simulink model "Los_path_old"  (R2023b)
settings: Solver=VariableStepAuto  StartTime=0.0  StopTime=200  RelTol=1e-3
values from neighbouring files (symbols this model uses):
  current = [0, 0, 0, 0]'    [Los_path_mat.m]
  deltah = 4    [Los_path_mat.m]
  depth_des = 0.5    [Los_path_mat.m]
  des_vel = [0.1, 0, 0, 0]'    [Kal_6Dpitch_mat.m]    (also in Los_path_mat.m)
  eta_init = [0.1, 0, 0, 0.7]'    [Los_path_mat.m]
  Kd_dep = (p + 2*damp*wn)*mv(3) + dv(3)    [Control_gains_mat.m]    (also in Los_path_mat.m = (p + 2*damp*wn)*mv(4) + dv(4))
  Kd_yaw = (p + 2*damp*wn)*mv(3) - dv(3)    [Los_path_mat.m]
  Ki_dep = p*(wn^2)*mv(3)    [Control_gains_mat.m]    (also in Los_path_mat.m = p*(wn^2)*mv(4))
  Ki_surge = wn^2 * mv(1)    [Control_gains_mat.m]    (also in Los_path_mat.m)
  Ki_yaw = p*(wn^2)*mv(3)    [Los_path_mat.m]
  Kp_dep = mv(3)*((wn^2) + 2*damp*p*wn)    [Control_gains_mat.m]    (also in Los_path_mat.m = mv(4)*((wn^2) + 2*damp*p*wn))
  Kp_surge = 2*damp*wn*mv(1) - dv(1)    [Control_gains_mat.m]    (also in Los_path_mat.m)
  Kp_yaw = mv(3)*((wn^2) + 2*damp*p*wn)    [Los_path_mat.m]
  speed0 = [0.1, 0, 0, 0]'    [Los_path_mat.m]    (also in Model_6Deq_mat.m = [0.1, 0, 0, 0, 0, 0]')
libraries: simulink x2
settings Model: Creator=fabio  LastModifiedBy=fabio

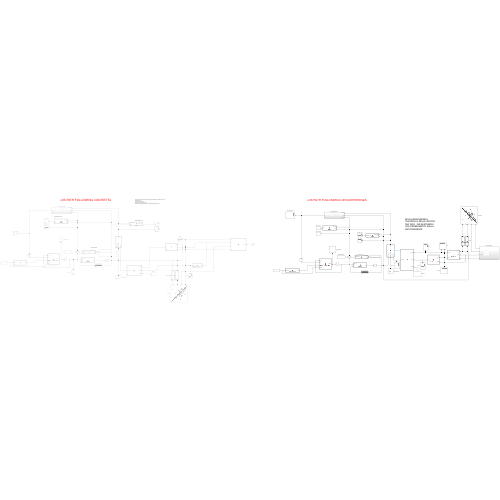
[thumbnail: Simulink's stored preview of the top-level diagram]
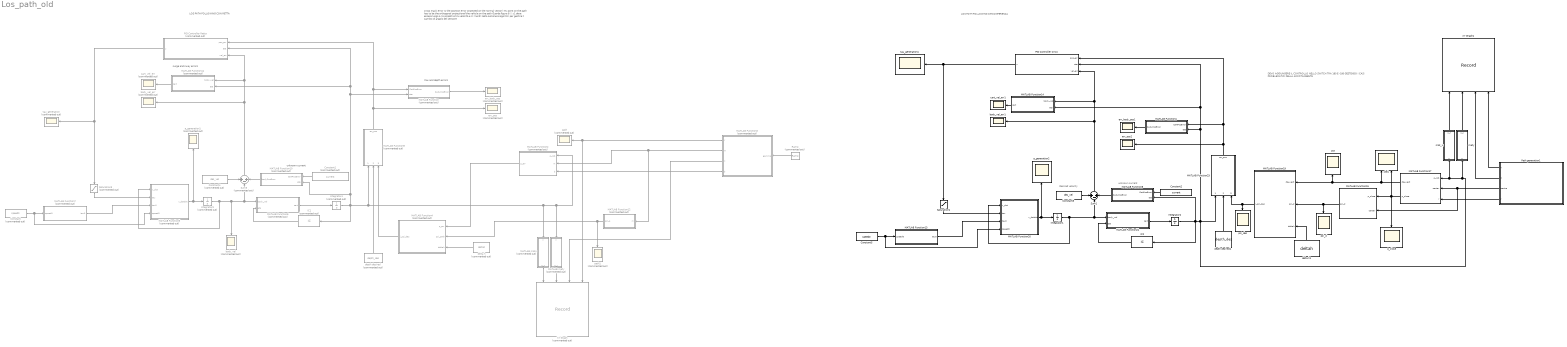
== system Los_path_old ==
  note: cross track error is the position error projected on the normal vector)
      | My point on the path has to be the orthogonal projectionof the vehicle on the path
      | Guarda figura 8 !!
      | y1 deve essere lungo a n1
      | psipath è tra velocità e Xi (nord)
      | Nella sezione 6 algoritm per gestire il cambio di angolo del sensore
  note: surge and sway errors
  note: Yaw and depth errors
  note: DEVO AGGIUNGERE IL CONTROLLO NELLO SWITCH TRA 180 E -180 GESTENDO I CASI PROBLEMATICI DELLA ARCOTANGENTE
  note: Desired velocity
  note: unknown current
  note: LOS PATH FOLLOWING CON RETTA
  note: unknown current
  note: LOS PATH FOLLOWING CIRCONFERENZA
  Constant : Constant  Commented=on  Value=speed0
  Constant1 : Constant  Commented=on  Value=current
  Constant2 : Constant  Value=current
  Constant3 : Constant  Value=des_vel
  Constant4 : Constant  Commented=on  Value=des_vel
  Constant5 : Constant  Value=speed0
  IC1 : InitialCondition  Commented=on  Value=eta_init
  IC2 : InitialCondition  Value=eta_init
  Integrator1 : Integrator
  Integrator2 : Integrator
  Integrator3 : Integrator  Commented=on
  Integrator4 : Integrator  Commented=on
  MATLAB Function : MATLAB Function  Commented=on  TreatAsAtomicUnit=on
  MATLAB Function1 : MATLAB Function  TreatAsAtomicUnit=on
  MATLAB Function10 : MATLAB Function  Commented=on  TreatAsAtomicUnit=on
  MATLAB Function11 : MATLAB Function  Commented=on  TreatAsAtomicUnit=on
  MATLAB Function12 : MATLAB Function  Commented=on  TreatAsAtomicUnit=on
  MATLAB Function13 : MATLAB Function  TreatAsAtomicUnit=on
  MATLAB Function14 : MATLAB Function  TreatAsAtomicUnit=on
  MATLAB Function15 : MATLAB Function  TreatAsAtomicUnit=on
  MATLAB Function17 : MATLAB Function  TreatAsAtomicUnit=on
  MATLAB Function19 : MATLAB Function  TreatAsAtomicUnit=on
  MATLAB Function2 : MATLAB Function  Commented=on  TreatAsAtomicUnit=on
  MATLAB Function20 : MATLAB Function  TreatAsAtomicUnit=on
  MATLAB Function21 : MATLAB Function  TreatAsAtomicUnit=on
  MATLAB Function23 : MATLAB Function  TreatAsAtomicUnit=on
  MATLAB Function3 : MATLAB Function  Commented=on  TreatAsAtomicUnit=on
  MATLAB Function4 : MATLAB Function  Commented=on  TreatAsAtomicUnit=on
  MATLAB Function5 : MATLAB Function  Commented=on  TreatAsAtomicUnit=on
  MATLAB Function6 : MATLAB Function  Commented=on  TreatAsAtomicUnit=on
  MATLAB Function7 : MATLAB Function  Commented=on  TreatAsAtomicUnit=on
  MATLAB Function8 : MATLAB Function  TreatAsAtomicUnit=on
  MATLAB Function9 : MATLAB Function  Commented=on  TreatAsAtomicUnit=on
  MATLAB matx : MATLAB Function  Commented=on  TreatAsAtomicUnit=on
  MATLAB maty : MATLAB Function  Commented=on  TreatAsAtomicUnit=on
  PID Controller Circo : Subsystem
  PID Controller Retta : Subsystem  Commented=on
  Path generation1 : Subsystem
  Ramp : simulink/Sources/Ramp  Commented=on  slope=1  start=0  InitialOutput=0
  Saturation1 : Saturate  UpperLimit=20000  LowerLimit=-20000
  Saturation3 : Saturate  Commented=on  UpperLimit=20000  LowerLimit=-20000
  Sum1 : Sum  Inputs=+-+
  Sum5 : Sum  Commented=on  Inputs=+-+
  XY Graph : Record  Commented=on  FileSettingsInternal="{\"entries\":[{\"content\":{\"excelSettings\":{\"content\":{},\"type\":\"Streamout.ExcelSettings\"}},\"type\":\"Streamout.FileSettingStorage\",\"uuid\":\"\"}],\"packageUris\":[\"http:\\/\\/schema.mathworks.com\\/mf0\\/streamout_blocks\\/R2020a\"],\"version\":\"1.0\"}"  Layout=[1 1]  SignalsInternal="{\"entries\":[{\"content\":{},\"type\":\"RecordBlkView.InputSignals\",\"uuid\":\"\"}],\"packageUris\":[\"http:\\/\\/schema.mathworks.com\\/mf0\\/streamout_blocks\\/R2020a\"],\"version\":\"1.0\"}"  VisualizationBindings="{\"xyplotplugin\":{\"info\":[{\"series\":[],\"subplotID\":1}]}}"  CompatibilityTag=XY
  XY Graph1 : Record  FileSettingsInternal="{\"entries\":[{\"content\":{\"excelSettings\":{\"content\":{},\"type\":\"Streamout.ExcelSettings\"}},\"type\":\"Streamout.FileSettingStorage\",\"uuid\":\"\"}],\"packageUris\":[\"http:\\/\\/schema.mathworks.com\\/mf0\\/streamout_blocks\\/R2020a\"],\"version\":\"1.0\"}"  Layout=[1 1]  SignalsInternal="{\"entries\":[{\"content\":{},\"type\":\"RecordBlkView.InputSignals\",\"uuid\":\"\"}],\"packageUris\":[\"http:\\/\\/schema.mathworks.com\\/mf0\\/streamout_blocks\\/R2020a\"],\"version\":\"1.0\"}"  VisualizationBindings="{\"xyplotplugin\":{\"info\":[{\"series\":[],\"subplotID\":1}]}}"  CompatibilityTag=XY
  a_generation1 : Scope  Commented=on
  a_generation2 : Scope
  body_vel : Scope  Commented=on
  body_vel_err : Scope  Commented=on
  body_vel_err1 : Scope
  cart_vel_err : Scope  Commented=on
  cart_vel_err1 : Scope
  cte : Scope
  cte1 : Scope  NumInputPorts=2
  delta h : Constant  Commented=on  Value=deltah
  delta h1 : Constant  Value=deltah
  depth desired : Constant  Commented=on  Value=depth_des
  depth desired1 : Constant  Value=depth_des
  err_body_pos : Scope  Commented=on
  err_body_pos1 : Scope
  err_pos : Scope  Commented=on
  err_pos2 : Scope
  mat_x : MATLAB Function  TreatAsAtomicUnit=on
  maty : MATLAB Function  TreatAsAtomicUnit=on
  p_close : Scope
  path : Scope  Commented=on
  path1 : Scope  Commented=on
  psi_d : Scope
  psi_des : Scope
  tau_generation : Scope  Commented=on
  tau_generation1 : Scope
  wires:
  PID Controller Retta/1(u) -> Saturation3/1, tau_generation/1
  Integrator3/1 -> body_vel/1, MATLAB Function6/1(body_vel), Sum5/2, MATLAB Function5/1(x_dot)
  Saturation3/1 -> MATLAB Function5/2(tau)
  MATLAB Function7/1(tau0) -> MATLAB Function5/3(tau0)
  MATLAB Function5/1(x_dotdot) -> Integrator3/1, a_generation1/1
  MATLAB Function6/1(cart) -> Integrator4/1
  IC1/1 -> MATLAB Function6/2(eta)
  MATLAB Function/1(bodyPosError) -> err_body_pos/1
  Sum5/1 -> PID Controller Retta/3(vel_err), MATLAB Function11/1(body_vel), body_vel_err/1
  Ramp/1 -> MATLAB Function3/1(gamma)
  MATLAB Function3/1(Y) -> path/1, XY Graph/4
  MATLAB Function3/2(m) -> MATLAB Function12/1(m), MATLAB Function2/2(m)
  MATLAB Function3/4(b) -> MATLAB Function2/3(b)
  Constant4/1 -> Sum5/1
  Integrator4/1 -> MATLAB Function9/1(p_pose_err), MATLAB Function2/1(p_rob), MATLAB maty/1(u), MATLAB matx/1(u), MATLAB Function/2(eta), PID Controller Retta/2(eta), MATLAB Function11/2(eta), MATLAB Function10/2(eta), IC1/1
  MATLAB Function4/1(i_psi_des) -> MATLAB Function9/3(psi_path)
  MATLAB Function9/1(err_pos) -> PID Controller Retta/1(pos_err), MATLAB Function/1(CartPosError), err_pos/1
  depth desired/1 -> MATLAB Function9/2(depth_des)
  MATLAB Function11/1(cart) -> cart_vel_err/1
  MATLAB matx/1(u_x) -> XY Graph/1
  MATLAB maty/1(u_y) -> XY Graph/2
  MATLAB Function3/3(X) -> XY Graph/3
  MATLAB Function12/1(psi_p) -> path1/1, MATLAB Function4/2(psi_path)
  MATLAB Function2/1(p_err) -> MATLAB Function4/1(p_err)
  delta h/1 -> MATLAB Function4/3(deltah)
  MATLAB Function21/1(cart) -> Integrator2/1
  Sum1/1 -> PID Controller Circo/3(vel_err), MATLAB Function14/1(body_vel), body_vel_err1/1
  depth desired1/1 -> MATLAB Function23/2(depth_des)
  MATLAB Function14/1(cart) -> cart_vel_err1/1
  MATLAB Function23/1(err_pos) -> err_pos2/1, PID Controller Circo/1(pos_err), MATLAB Function1/1(CartPosError)
  Integrator1/1 -> MATLAB Function21/1(body_vel), Sum1/2, MATLAB Function20/1(x_dot)
  Constant3/1 -> Sum1/1
  MATLAB Function20/1(x_dotdot) -> Integrator1/1, a_generation2/1
  Integrator2/1 -> MATLAB Function8/2(eta), maty/1(u), mat_x/1(u), MATLAB Function17/1(p_rob), MATLAB Function14/2(eta), PID Controller Circo/2(eta), MATLAB Function1/2(eta), MATLAB Function23/1(p_pose_err), IC2/1
  MATLAB Function19/1(i_psi_des) -> MATLAB Function23/3(psi_path), psi_des/1
  MATLAB Function1/1(bodyPosError) -> err_body_pos1/1
  Saturation1/1 -> MATLAB Function20/2(tau)
  PID Controller Circo/1(u) -> Saturation1/1, tau_generation1/1
  IC2/1 -> MATLAB Function21/2(eta)
  Path generation1/3(centre) -> MATLAB Function15/2(center), MATLAB Function17/2(center)
  Path generation1/4(r) -> MATLAB Function17/3(r)
  MATLAB Function17/2(p_close) -> p_close/1, MATLAB Function15/1(p_close), cte1/2
  MATLAB Function15/1(psi_d) -> psi_d/1, MATLAB Function19/2(psi_d)
  MATLAB Function17/1(cte_vect) -> MATLAB Function19/1(cte_vect), cte/1, cte1/1
  delta h1/1 -> MATLAB Function19/3(deltah)
  Path generation1/2(X) -> XY Graph1/3
  Path generation1/1(Y) -> XY Graph1/4
  mat_x/1(u_x) -> XY Graph1/1
  maty/1(u_y) -> XY Graph1/2
  Constant2/1 -> MATLAB Function8/1(CartPosError)
  MATLAB Function8/1(bodyPosError) -> Sum1/3
  MATLAB Function10/1(bodyPosError) -> Sum5/3
  Constant1/1 -> MATLAB Function10/1(CartPosError)
  Constant/1 -> MATLAB Function5/4(speed0), MATLAB Function7/1(speed0)
  MATLAB Function13/1(tau0) -> MATLAB Function20/3(tau0)
  Constant5/1 -> MATLAB Function20/4(speed0), MATLAB Function13/1(speed0)

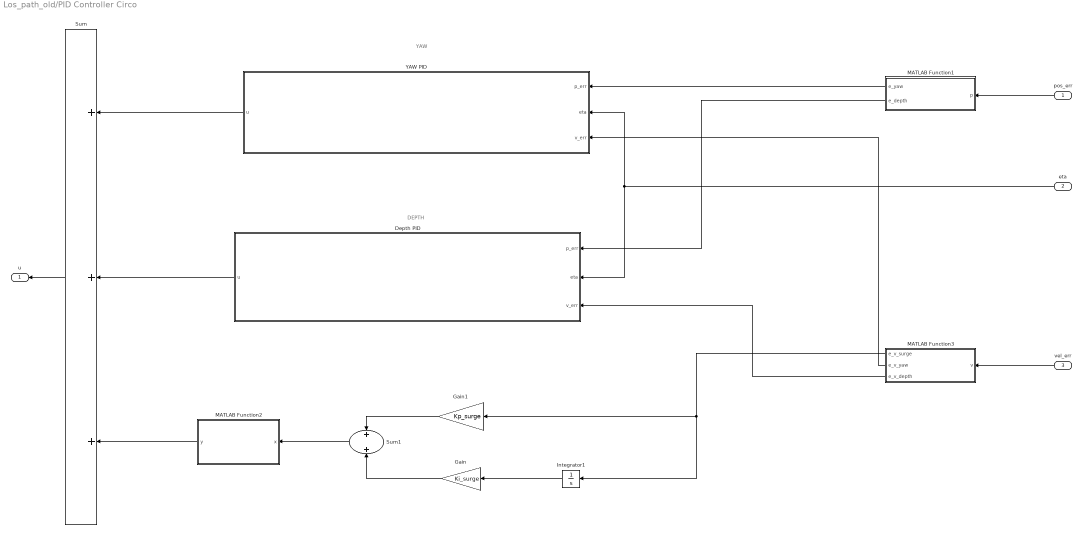
== system Los_path_old/PID Controller Circo ==
  note: YAW
  note: DEPTH
  pos_err : Inport
  eta : Inport  Port=2
  vel_err : Inport  Port=3
  Depth PID : Subsystem
  Gain : Gain  Gain=Ki_surge
  Gain1 : Gain  Gain=Kp_surge
  Integrator1 : Integrator
  MATLAB Function1 : MATLAB Function  TreatAsAtomicUnit=on
  MATLAB Function2 : MATLAB Function  TreatAsAtomicUnit=on
  MATLAB Function3 : MATLAB Function  TreatAsAtomicUnit=on
  Sum : Sum  Inputs=+++
  Sum1 : Sum
  YAW PID : Subsystem
  u : Outport
  wires:
  vel_err/1 -> MATLAB Function3/1(v)
  pos_err/1 -> MATLAB Function1/1(p)
  MATLAB Function1/2(e_depth) -> Depth PID/1(p_err)
  Integrator1/1 -> Gain/1
  Gain1/1 -> Sum1/1
  Sum/1 -> u/1
  YAW PID/1(u) -> Sum/1
  MATLAB Function1/1(e_yaw) -> YAW PID/1(p_err)
  Depth PID/1(u) -> Sum/2
  Gain/1 -> Sum1/2
  MATLAB Function3/1(e_v_surge) -> Gain1/1, Integrator1/1
  MATLAB Function3/2(e_v_yaw) -> YAW PID/3(v_err)
  MATLAB Function3/3(e_v_depth) -> Depth PID/3(v_err)
  Sum1/1 -> MATLAB Function2/1(x)
  eta/1 -> YAW PID/2(eta), Depth PID/2(eta)
  MATLAB Function2/1(y) -> Sum/3

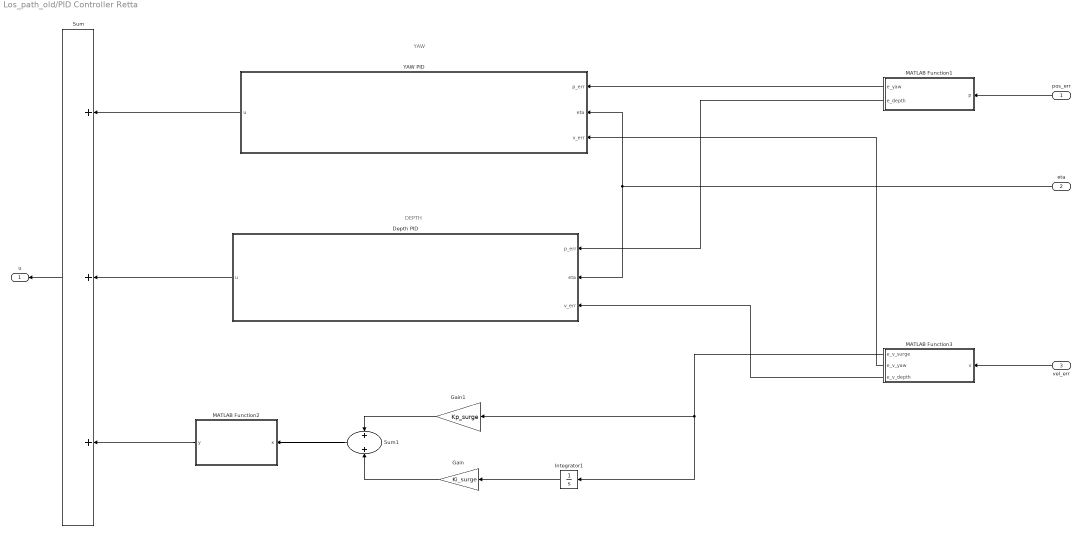
== system Los_path_old/PID Controller Retta ==
  note: DEPTH
  note: YAW
  pos_err : Inport
  eta : Inport  Port=2
  vel_err : Inport  Port=3
  Depth PID : Subsystem
  Gain : Gain  Gain=Ki_surge
  Gain1 : Gain  Gain=Kp_surge
  Integrator1 : Integrator
  MATLAB Function1 : MATLAB Function  TreatAsAtomicUnit=on
  MATLAB Function2 : MATLAB Function  TreatAsAtomicUnit=on
  MATLAB Function3 : MATLAB Function  TreatAsAtomicUnit=on
  Sum : Sum  Inputs=+++
  Sum1 : Sum
  YAW PID : Subsystem
  u : Outport
  wires:
  eta/1 -> YAW PID/2(eta), Depth PID/2(eta)
  Integrator1/1 -> Gain/1
  Sum1/1 -> MATLAB Function2/1(x)
  Sum/1 -> u/1
  MATLAB Function3/1(e_v_surge) -> Gain1/1, Integrator1/1
  Depth PID/1(u) -> Sum/2
  YAW PID/1(u) -> Sum/1
  pos_err/1 -> MATLAB Function1/1(p)
  vel_err/1 -> MATLAB Function3/1(v)
  MATLAB Function1/1(e_yaw) -> YAW PID/1(p_err)
  MATLAB Function1/2(e_depth) -> Depth PID/1(p_err)
  MATLAB Function2/1(y) -> Sum/3
  Gain1/1 -> Sum1/1
  Gain/1 -> Sum1/2
  MATLAB Function3/2(e_v_yaw) -> YAW PID/3(v_err)
  MATLAB Function3/3(e_v_depth) -> Depth PID/3(v_err)

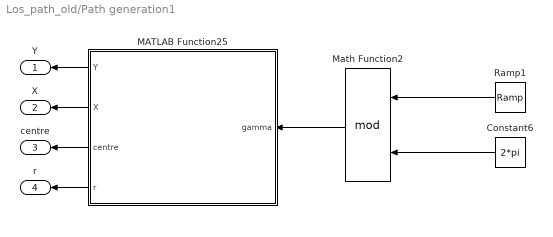
== system Los_path_old/Path generation1 ==
  Constant6 : Constant  Value=2*pi
  MATLAB Function25 : MATLAB Function  TreatAsAtomicUnit=on
  Math Function2 : Math  Operator=mod  SignedPower=on  RndMeth=Zero
  Ramp1 : simulink/Sources/Ramp  slope=0.5  start=0  InitialOutput=0
  Y : Outport
  X : Outport  Port=2
  centre : Outport  Port=3
  r : Outport  Port=4
  wires:
  Ramp1/1 -> Math Function2/1
  Math Function2/1 -> MATLAB Function25/1(gamma)
  Constant6/1 -> Math Function2/2
  MATLAB Function25/4(r) -> r/1
  MATLAB Function25/3(centre) -> centre/1
  MATLAB Function25/1(Y) -> Y/1
  MATLAB Function25/2(X) -> X/1

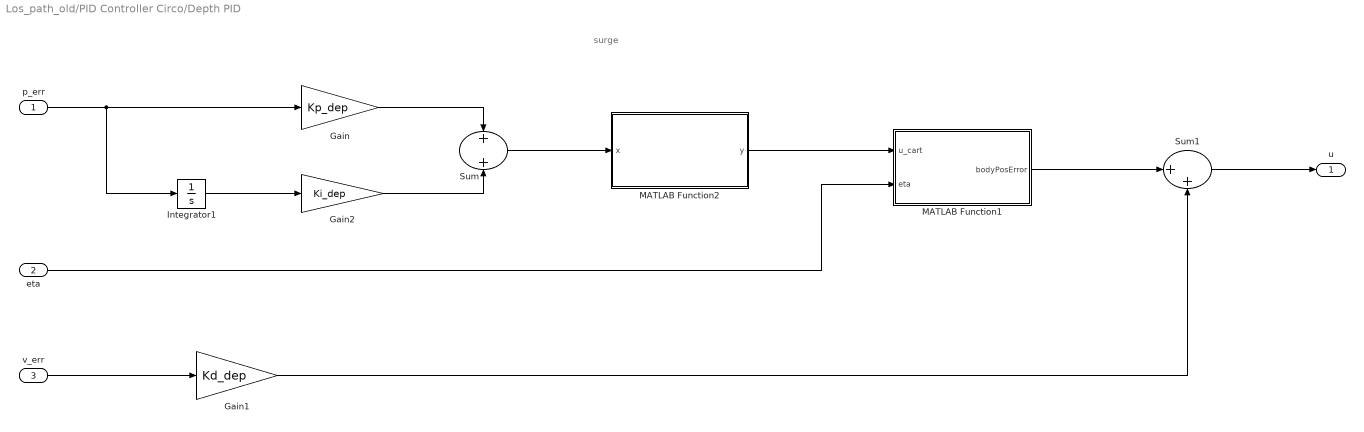
== system Los_path_old/PID Controller Circo/Depth PID ==
  note: surge
  p_err : Inport
  eta : Inport  Port=2
  v_err : Inport  Port=3
  Gain : Gain  Gain=Kp_dep
  Gain1 : Gain  Gain=Kd_dep
  Gain2 : Gain  Gain=Ki_dep
  Integrator1 : Integrator
  MATLAB Function1 : MATLAB Function  TreatAsAtomicUnit=on
  MATLAB Function2 : MATLAB Function  TreatAsAtomicUnit=on
  Sum : Sum
  Sum1 : Sum  Inputs=|++
  u : Outport
  wires:
  Sum1/1 -> u/1
  Sum/1 -> MATLAB Function2/1(x)
  Gain1/1 -> Sum1/2
  p_err/1 -> Integrator1/1, Gain/1
  MATLAB Function1/1(bodyPosError) -> Sum1/1
  MATLAB Function2/1(y) -> MATLAB Function1/1(u_cart)
  Gain/1 -> Sum/1
  v_err/1 -> Gain1/1
  eta/1 -> MATLAB Function1/2(eta)
  Integrator1/1 -> Gain2/1
  Gain2/1 -> Sum/2

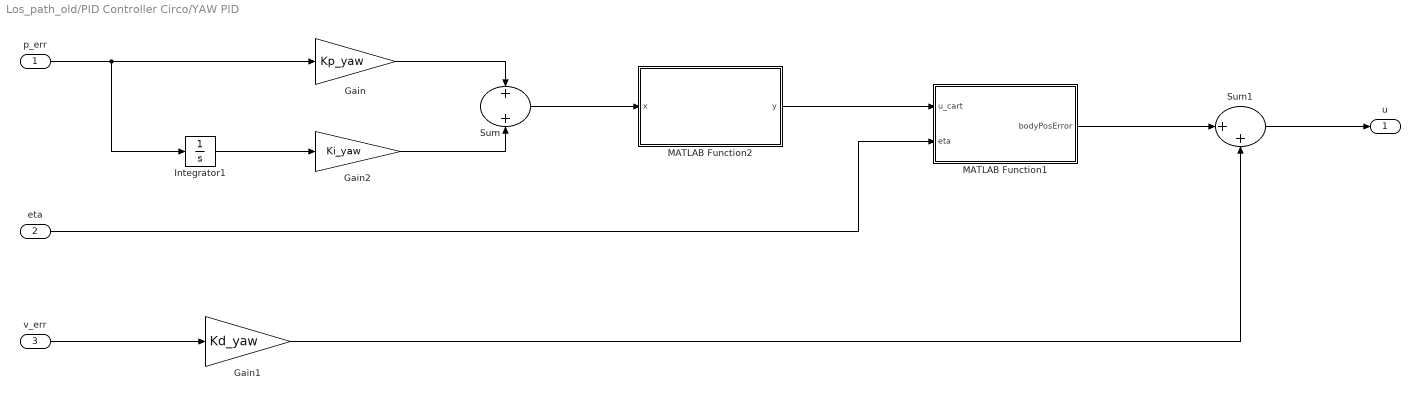
== system Los_path_old/PID Controller Circo/YAW PID ==
  p_err : Inport
  eta : Inport  Port=2
  v_err : Inport  Port=3
  Gain : Gain  Gain=Kp_yaw
  Gain1 : Gain  Gain=Kd_yaw
  Gain2 : Gain  Gain=Ki_yaw
  Integrator1 : Integrator
  MATLAB Function1 : MATLAB Function  TreatAsAtomicUnit=on
  MATLAB Function2 : MATLAB Function  TreatAsAtomicUnit=on
  Sum : Sum
  Sum1 : Sum  Inputs=|++
  u : Outport
  wires:
  p_err/1 -> Integrator1/1, Gain/1
  Integrator1/1 -> Gain2/1
  Gain2/1 -> Sum/2
  Gain/1 -> Sum/1
  Sum/1 -> MATLAB Function2/1(x)
  MATLAB Function2/1(y) -> MATLAB Function1/1(u_cart)
  eta/1 -> MATLAB Function1/2(eta)
  MATLAB Function1/1(bodyPosError) -> Sum1/1
  Gain1/1 -> Sum1/2
  v_err/1 -> Gain1/1
  Sum1/1 -> u/1

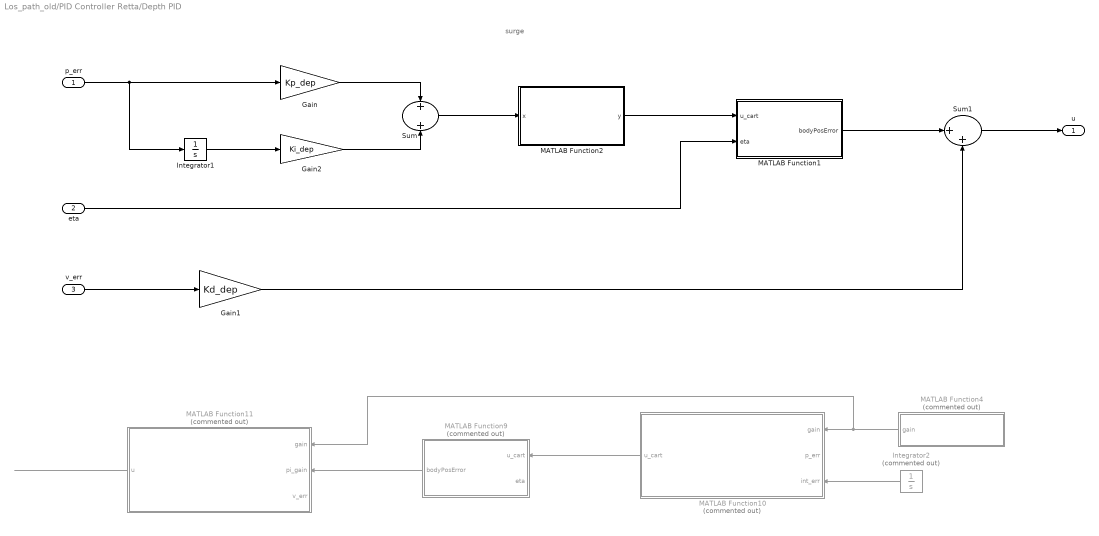
== system Los_path_old/PID Controller Retta/Depth PID ==
  note: surge
  p_err : Inport
  eta : Inport  Port=2
  v_err : Inport  Port=3
  Gain : Gain  Gain=Kp_dep
  Gain1 : Gain  Gain=Kd_dep
  Gain2 : Gain  Gain=Ki_dep
  Integrator1 : Integrator
  Integrator2 : Integrator  Commented=on
  MATLAB Function1 : MATLAB Function  TreatAsAtomicUnit=on
  MATLAB Function10 : MATLAB Function  Commented=on  TreatAsAtomicUnit=on
  MATLAB Function11 : MATLAB Function  Commented=on  TreatAsAtomicUnit=on
  MATLAB Function2 : MATLAB Function  TreatAsAtomicUnit=on
  MATLAB Function4 : MATLAB Function  Commented=on  TreatAsAtomicUnit=on
  MATLAB Function9 : MATLAB Function  Commented=on  TreatAsAtomicUnit=on
  Sum : Sum
  Sum1 : Sum  Inputs=|++
  u : Outport
  wires:
  MATLAB Function10/1(u_cart) -> MATLAB Function9/1(u_cart)
  Integrator2/1 -> MATLAB Function10/3(int_err)
  MATLAB Function4/1(gain) -> MATLAB Function11/1(gain), MATLAB Function10/1(gain)
  MATLAB Function9/1(bodyPosError) -> MATLAB Function11/2(pi_gain)
  MATLAB Function11/1(u) -> ?
  Sum1/1 -> u/1
  Sum/1 -> MATLAB Function2/1(x)
  Gain1/1 -> Sum1/2
  p_err/1 -> Integrator1/1, Gain/1
  MATLAB Function1/1(bodyPosError) -> Sum1/1
  MATLAB Function2/1(y) -> MATLAB Function1/1(u_cart)
  Gain/1 -> Sum/1
  v_err/1 -> Gain1/1
  eta/1 -> MATLAB Function1/2(eta)
  Integrator1/1 -> Gain2/1
  Gain2/1 -> Sum/2

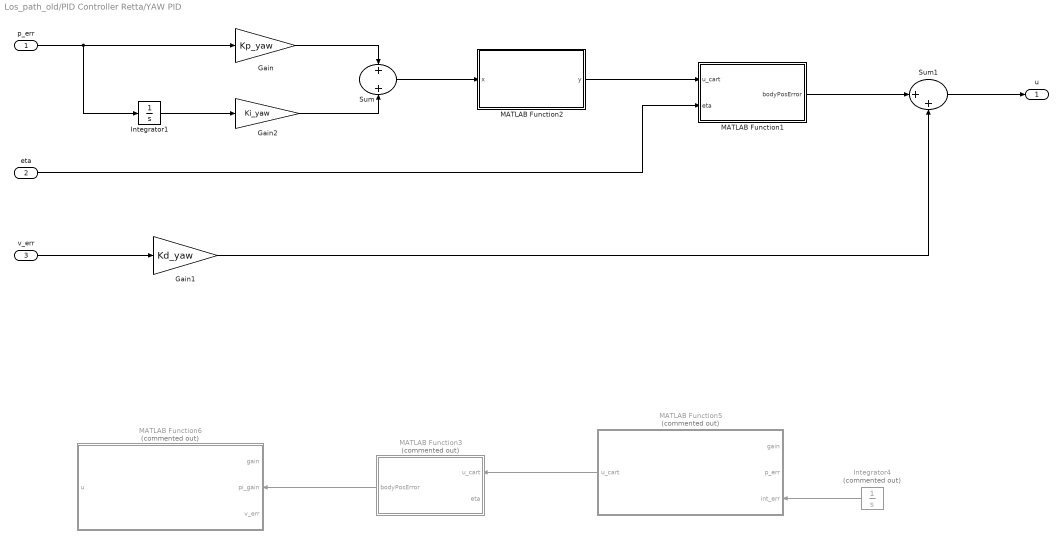
== system Los_path_old/PID Controller Retta/YAW PID ==
  p_err : Inport
  eta : Inport  Port=2
  v_err : Inport  Port=3
  Gain : Gain  Gain=Kp_yaw
  Gain1 : Gain  Gain=Kd_yaw
  Gain2 : Gain  Gain=Ki_yaw
  Integrator1 : Integrator
  Integrator4 : Integrator  Commented=on
  MATLAB Function1 : MATLAB Function  TreatAsAtomicUnit=on
  MATLAB Function2 : MATLAB Function  TreatAsAtomicUnit=on
  MATLAB Function3 : MATLAB Function  Commented=on  TreatAsAtomicUnit=on
  MATLAB Function5 : MATLAB Function  Commented=on  TreatAsAtomicUnit=on
  MATLAB Function6 : MATLAB Function  Commented=on  TreatAsAtomicUnit=on
  Sum : Sum
  Sum1 : Sum  Inputs=|++
  u : Outport
  wires:
  Integrator4/1 -> MATLAB Function5/3(int_err)
  MATLAB Function3/1(bodyPosError) -> MATLAB Function6/2(pi_gain)
  MATLAB Function5/1(u_cart) -> MATLAB Function3/1(u_cart)
  p_err/1 -> Integrator1/1, Gain/1
  Integrator1/1 -> Gain2/1
  Gain2/1 -> Sum/2
  Gain/1 -> Sum/1
  Sum/1 -> MATLAB Function2/1(x)
  MATLAB Function2/1(y) -> MATLAB Function1/1(u_cart)
  eta/1 -> MATLAB Function1/2(eta)
  MATLAB Function1/1(bodyPosError) -> Sum1/1
  Gain1/1 -> Sum1/2
  v_err/1 -> Gain1/1
  Sum1/1 -> u/1

== matlab function Los_path_old/MATLAB matx ==
  data: u input; u_x output
function u_x = Conditioning(u)
    u_x = u(1);
end

== matlab function Los_path_old/MATLAB Function6 ==
  data: cart output; body_vel input; eta input
function cart = mapping(body_vel, eta)
    Jacobian = eye(4);
    angle = eta(3);
    Jacobian(1:2, 1:2) = [cos(angle), -sin(angle);
                          sin(angle), cos(angle)];
    cart = Jacobian * body_vel;
end

== matlab function Los_path_old/MATLAB Function7 ==
  data: tau0 output; speed0 input
function tau0 = tau0Computation(speed0)
    % updated to medusa model
    m = 30;
    I = 4.14;
    g = 9.81;
    WB = -0.8339; % Buoyancy

    % Added mass
    tau_a = [-25; -2.325; -8.690; -19.4311]; % kl_dot

    % Restoring forces
    tau_r = [-0.2; -55.117; -4.14; 33.6804]; % kl

    % Hydrodynamic forces
    tau_d = [-19.5; -147.9; -6.23; -89.4105]; % kl_modl

    % Virtual mass
    mv = [m; m; I; m] - tau_a;

    % Dissatipative forces
    dv = -tau_r - 2*tau_d .* abs(speed0);
    
    % tau0 computation
    tau0 = zeros(4,1);
    tau0(1) = dv(1)*speed0(1) - mv(2)*speed0(2)*speed0(3);
    tau0(2) = 0; % can do also the equations
    tau0(3) = dv(3)*speed0(3) - (mv(1) - mv(2))*speed0(1)*speed0(2);
    tau0(4) = -dv(4)*speed0(4) - WB;
end

== matlab function Los_path_old/MATLAB Function14 ==
  data: cart output; body_vel input; eta input
function cart = mapping(body_vel, eta)
    cart = zeros(4,1);
    Jacobian = eye(4);
    angle = eta(3);
    Jacobian(1:2, 1:2) = [cos(angle), -sin(angle);
                          sin(angle), cos(angle)];
    cart = Jacobian * body_vel;
end

== matlab function Los_path_old/MATLAB maty ==
  data: u input; u_y output
function u_y = Conditioning(u)
    u_y = u(2);
end

== matlab function Los_path_old/MATLAB Function15 ==
  data: p_close input; psi_d output; center input
function psi_d = trajectory_orientation(p_close, center)
    dist = p_close - center;
    % Considerando il vettore tangente per avere psi_p
    theta_r = atan2(-dist(2), dist(1));
    % Dovrebbe corrispondere ad angolo tra tangente e asse x positivo
    psi_d = theta_r + pi/2;
end

== matlab function Los_path_old/MATLAB Function ==
  data: CartPosError input; bodyPosError output; eta input
function bodyPosError = Rotation(CartPosError, eta)
    angle = eta(3);
    bodyPosError = zeros(4,1);
    rot = [cos(angle), -sin(angle)
            sin(angle), cos(angle)];

    bodyPosError(1:2) = rot' * CartPosError(1:2);
    bodyPosError(3:4) = CartPosError(3:4);
end

== matlab function Los_path_old/maty ==
  data: u input; u_y output
function u_y = Conditioning(u)
    u_y = u(2);
end

== matlab function Los_path_old/MATLAB Function17 ==
  data: cte_vect output; p_rob input; center input; r input; p_close output
function [cte_vect, p_close] = ClosestPoint(p_rob, center, r)
    p_close = zeros(2,1);
    d = sqrt((p_rob(1) - center(1))^2 + (p_rob(2) - center(2))^2);
    lamda = r / d;
    p_close(1) = center(1) + lamda * (p_rob(1) - center(1));
    p_close(2) = center(2) + lamda * (p_rob(2) - center(2));
    cte_vect = p_rob(1:2) - p_close;
end

== matlab function Los_path_old/Path generation1/MATLAB Function25 ==
  data: Y output; X output; centre output; r output; gamma input
function [Y, X, centre, r] = path(gamma)
    % gamma is the theta
    centre = [4,4];
    r = 3;
    X = r * cos(gamma) + centre(1);
    Y = r * sin(gamma) + centre(2);
end

== matlab function Los_path_old/MATLAB Function19 ==
  data: cte_vect input; i_psi_des output; psi_d input; deltah input
function i_psi_des = Error(cte_vect, psi_d, deltah)
    % attenzione: Non vero cross ttrack error che vorrebbe solo distanza
    % lungo la verticale
    % distanza perpendicolare dal robot alla tangente della circonferenza.
    y1 = sign(cte_vect(2)) * sqrt((cte_vect(1))^2 + (cte_vect(2)^2));
    i_psi_des = psi_d + atan2(-y1 , deltah);
end

== matlab function Los_path_old/MATLAB Function20 ==
  data: x_dot input; tau input; tau0 input; x_dotdot output; speed0 input
function x_dotdot = vehicle_dynamics_matrix(x_dot, tau, tau0, speed0)
    % updated to medusa model
    m = 30;
    I = 4.14;

    % Added mass
    tau_a = [-25; -2.325; -8.690; -19.4311]; % kl_dot

    % Restoring forces
    tau_r = [-0.2; -55.117; -4.14; 33.6804]; % kl

    % Hydrodynamic forces
    tau_d = [-19.5; -147.9; -6.23; -89.4105]; % kl_modl

    % Virtual mass
    mv = [m; m; I; m] - tau_a;

    % Dissatipative forces
    dv = -tau_r - 2*tau_d .* abs(speed0);

    delta = x_dot - speed0;

    % Accelerations
    % 3 DOF MODEL Linearized
    x_dotdot = zeros(4,1);
    tau(2) = 0;
    x_dotdot(1) = (tau(1) - tau0(1) - dv(1)*delta(1) + mv(2)*speed0(2)*delta(3) + mv(2)*speed0(3)*delta(2)) / mv(1); 
    x_dotdot(2) = (tau(2) - tau0(2) - dv(2)*delta(2) - mv(1)*speed0(1)*delta(3) - mv(1)*speed0(3)*delta(1)) / mv(2);
    x_dotdot(3) = (tau(3) - tau0(3) - dv(3)*delta(3) + (mv(1) - mv(2))*speed0(1)*delta(2) + (mv(1) - mv(2))*speed0(2)*delta(1)) / mv(3);
    % Considering also depth (heavy)
    x_dotdot(4) = (tau(4) - tau0(4) + dv(4)*delta(4)) / mv(4);
end

== matlab function Los_path_old/MATLAB Function21 ==
  data: cart output; body_vel input; eta input
function cart = mapping(body_vel, eta)
    cart = zeros(4,1);
    Jacobian = eye(4);
    angle = eta(3);
    Jacobian(1:2, 1:2) = [cos(angle), -sin(angle);
                          sin(angle), cos(angle)];
    cart = Jacobian * body_vel;
end

== matlab function Los_path_old/MATLAB Function13 ==
  data: tau0 output; speed0 input
function tau0 = tau0Computation(speed0)
    % updated to medusa model
    m = 30;
    I = 4.14;
    g = 9.81;
    WB = -0.8339; % Buoyancy

    % Added mass
    tau_a = [-25; -2.325; -8.690; -19.4311]; % kl_dot

    % Restoring forces
    tau_r = [-0.2; -55.117; -4.14; 33.6804]; % kl

    % Hydrodynamic forces
    tau_d = [-19.5; -147.9; -6.23; -89.4105]; % kl_modl

    % Virtual mass
    mv = [m; m; I; m] - tau_a;

    % Dissatipative forces
    dv = -tau_r - 2*tau_d .* abs(speed0);
    
    % tau0 computation
    tau0 = zeros(4,1);
    tau0(1) = dv(1)*speed0(1) - mv(2)*speed0(2)*speed0(3);
    tau0(2) = 0; % can do also the equations
    tau0(3) = dv(3)*speed0(3) - (mv(1) - mv(2))*speed0(1)*speed0(2);
    tau0(4) = -dv(4)*speed0(4) - WB;
end

== matlab function Los_path_old/MATLAB Function23 ==
  data: p_pose_err input; depth_des input; err_pos output; psi_path input
function err_pos = psi_err(p_pose_err, depth_des, psi_path)
    err_pos = zeros(4,1);
    err_pos(3) = psi_path - p_pose_err(3);
    err_pos(4) = depth_des - p_pose_err(4);
end

== matlab function Los_path_old/mat_x ==
  data: u input; u_x output
function u_x = Conditioning(u)
    u_x = u(1);
end

== matlab function Los_path_old/MATLAB Function11 ==
  data: cart output; body_vel input; eta input
function cart = mapping(body_vel, eta)
    cart = zeros(4,1);
    Jacobian = eye(4);
    angle = eta(3);
    Jacobian(1:2, 1:2) = [cos(angle), -sin(angle);
                          sin(angle), cos(angle)];
    cart = Jacobian * body_vel;
end

== matlab function Los_path_old/PID Controller Circo/Depth PID/MATLAB Function2 ==
  data: x input; y output
function y = Cond(x)
    y = zeros(4,1);
    y(4) = x;
end

== matlab function Los_path_old/MATLAB Function8 ==
  data: CartPosError input; bodyPosError output; eta input
function bodyPosError = Rotation(CartPosError, eta)
    angle = eta(3);
    bodyPosError = zeros(4,1);
    rot = [cos(angle), -sin(angle)
            sin(angle), cos(angle)];

    bodyPosError(1:2) = rot' * CartPosError(1:2);
    bodyPosError(3:4) = CartPosError(3:4);
end

== matlab function Los_path_old/MATLAB Function10 ==
  data: CartPosError input; bodyPosError output; eta input
function bodyPosError = Rotation(CartPosError, eta)
    angle = eta(3);
    bodyPosError = zeros(4,1);
    rot = [cos(angle), -sin(angle)
            sin(angle), cos(angle)];

    bodyPosError(1:2) = rot' * CartPosError(1:2);
    bodyPosError(3:4) = CartPosError(3:4);
end

== matlab function Los_path_old/PID Controller Retta/YAW PID/MATLAB Function1 ==
  data: u_cart input; bodyPosError output; eta input
function bodyPosError = Rotation(u_cart, eta)
    angle = eta(3);
    bodyPosError = zeros(4,1);
    rot = [cos(angle), -sin(angle)
            sin(angle), cos(angle)];

    bodyPosError(1:2) = rot' * u_cart(1:2);
    bodyPosError(3:4) = u_cart(3:4);
end

== matlab function Los_path_old/PID Controller Retta/YAW PID/MATLAB Function2 ==
  data: x input; y output
function y = Cond(x)
    y = zeros(4,1);
    y(3) = x;
end

== matlab function Los_path_old/PID Controller Retta/Depth PID/MATLAB Function4 ==
  data: gain output
function gain = gainComputation()
    m = 30;
    I = 4.14;
    wn = 0.2;
    damp = 0.6;
    p = -10;
    
    % x initial
    speed0 = [0.1, 0, 0, 0]';

    % Added mass
    tau_a = [-25; -2.325; -8.690; -19.4311]; % kl_dot

    % Restoring forces
    tau_r = [-0.2; -55.117; -4.14; 33.6804]; % kl

    % Hydrodynamic forces
    tau_d = [-19.5; -147.9; -6.23; -89.4105]; % kl_modl (era -89...

    % Virtual mass
    mv = [m; m; I; m] - tau_a;

    % Dissatipative forces
    dv = -tau_r - 2*tau_d .* abs(speed0);
    %% DEPTH (pid)
    Kd_dep = (p + 2*damp*wn)*mv(4) + dv(4);
    Kp_dep = mv(4)*((wn^2) + 2*damp*p*wn);
    Ki_dep = p*(wn^2)*mv(4);
    %% TOTAL CONTROLLERS
    gain = [Kd_dep, Kp_dep, Ki_dep]; %kd, kp, ki
end

== matlab function Los_path_old/PID Controller Retta/Depth PID/MATLAB Function10 ==
  data: gain input; u_cart output; p_err input; int_err input
function u_cart = PI(gain, p_err, int_err)
    u_cart = zeros(4,1);
    u_cart(4) = gain(2) * p_err + gain(3) * int_err;
end

== matlab function Los_path_old/PID Controller Retta/YAW PID/MATLAB Function3 ==
  data: u_cart input; bodyPosError output; eta input
function bodyPosError = Rotation(u_cart, eta)
    angle = eta(3);
    bodyPosError = zeros(4,1);
    rot = [cos(angle), -sin(angle)
            sin(angle), cos(angle)];

    bodyPosError(1:2) = rot' * u_cart(1:2);
    bodyPosError(3:4) = u_cart(3:4);
end

== matlab function Los_path_old/PID Controller Retta/Depth PID/MATLAB Function11 ==
  data: gain input; u output; pi_gain input; v_err input
function u = PID(gain, pi_gain, v_err)
    u = zeros(4,1);
    u(4) = gain(1) * v_err + pi_gain(4);
end

== matlab function Los_path_old/PID Controller Retta/YAW PID/MATLAB Function5 ==
  data: gain input; u_cart output; p_err input; int_err input
function u_cart = PI(gain, p_err, int_err)
    u_cart = zeros(4,1);
    u_cart(3) = gain(2) * p_err + gain(3) * int_err;
end

== matlab function Los_path_old/MATLAB Function3 ==
  data: gamma input; Y output; m output; X output; b output
function [Y, m, X, b] = path(gamma)
    % North (x) East(y) inertial frame definition
    % p(gamma) = p0 + gamma * d_unitario
    % gamma is my x, the arc length
    X = gamma;
    m = 0.4;
    b = 1;
    Y = m*X + b;                                   
end

== matlab function Los_path_old/PID Controller Retta/YAW PID/MATLAB Function6 ==
  data: gain input; u output; pi_gain input; v_err input
function u = PID(gain, pi_gain, v_err)
    u = zeros(4,1);
    u(3) = gain(1) * v_err + pi_gain(3);
end

== matlab function Los_path_old/PID Controller Retta/Depth PID/MATLAB Function9 ==
  data: u_cart input; bodyPosError output; eta input
function bodyPosError = Rotation(u_cart, eta)
    angle = eta(3);
    bodyPosError = zeros(4,1);
    rot = [cos(angle), -sin(angle)
            sin(angle), cos(angle)];

    bodyPosError(1:2) = rot' * u_cart(1:2);
    bodyPosError(3:4) = u_cart(3:4);
end

== matlab function Los_path_old/PID Controller Circo/MATLAB Function1 ==
  data: e_yaw output; p input; e_depth output
function [e_yaw, e_depth] = Deviator(p)
    e_yaw = p(3);
    e_depth = p(4);
end

== matlab function Los_path_old/PID Controller Retta/MATLAB Function1 ==
  data: e_yaw output; p input; e_depth output
function [e_yaw, e_depth] = Deviator(p)
    e_yaw = p(3);
    e_depth = p(4);
end

== matlab function Los_path_old/PID Controller Retta/MATLAB Function3 ==
  data: e_v_surge output; v input; e_v_yaw output; e_v_depth output
function [e_v_surge, e_v_yaw, e_v_depth] = Deviator(v)
    e_v_surge = v(1);
    e_v_yaw = v(3);
    e_v_depth = v(4);
end

== matlab function Los_path_old/PID Controller Retta/Depth PID/MATLAB Function1 ==
  data: u_cart input; bodyPosError output; eta input
function bodyPosError = Rotation(u_cart, eta)
    angle = eta(3);
    bodyPosError = zeros(4,1);
    rot = [cos(angle), -sin(angle)
            sin(angle), cos(angle)];

    bodyPosError(1:2) = rot' * u_cart(1:2);
    bodyPosError(3:4) = u_cart(3:4);
end

== matlab function Los_path_old/PID Controller Retta/Depth PID/MATLAB Function2 ==
  data: x input; y output
function y = Cond(x)
    y = zeros(4,1);
    y(4) = x;
end

== matlab function Los_path_old/PID Controller Retta/MATLAB Function2 ==
  data: x input; y output
function y = Cond(x)
    y = zeros(4,1);
    y(1) = x;
end

== matlab function Los_path_old/PID Controller Circo/MATLAB Function2 ==
  data: x input; y output
function y = Cond(x)
    y = zeros(4,1);
    y(1) = x;
end

== matlab function Los_path_old/PID Controller Circo/MATLAB Function3 ==
  data: e_v_surge output; v input; e_v_yaw output; e_v_depth output
function [e_v_surge, e_v_yaw, e_v_depth] = Deviator(v)
    e_v_surge = v(1);
    e_v_yaw = v(3);
    e_v_depth = v(4);
end

== matlab function Los_path_old/PID Controller Circo/YAW PID/MATLAB Function1 ==
  data: u_cart input; bodyPosError output; eta input
function bodyPosError = Rotation(u_cart, eta)
    angle = eta(3);
    bodyPosError = zeros(4,1);
    rot = [cos(angle), -sin(angle)
            sin(angle), cos(angle)];

    bodyPosError(1:2) = rot' * u_cart(1:2);
    bodyPosError(3:4) = u_cart(3:4);
end

== matlab function Los_path_old/PID Controller Circo/YAW PID/MATLAB Function2 ==
  data: x input; y output
function y = Cond(x)
    y = zeros(4,1);
    y(3) = x;
end

== matlab function Los_path_old/MATLAB Function2 ==
  data: p_err output; p_rob input; m input; b input
function p_err = ClosestPoint(p_rob, m, b)
    p_close = zeros(2,1);
    p_close(1) = (p_rob(1) + m*(p_rob(2) - b)) / (1 + m^2);
    p_close(2) = m*p_close(1) + b;
    % error is the difference between p - pd in inertia frame trasformed
    % then in path frame
    p_err = p_rob(1:2) - p_close;
end

== matlab function Los_path_old/MATLAB Function4 ==
  data: p_err input; i_psi_des output; psi_path input; deltah input
function i_psi_des = Error(p_err, psi_path, deltah)
    % depth control
    % attenzione: y1 deve essere lungo a n1
    % giustamente il punto più vicino è gia perpendicolare (parallelo a n)
    % y1 = p_err(2);
    y1 = sign(p_err(2)) * sqrt((p_err(1))^2 + (p_err(2)^2));
    i_psi_des = psi_path + atan2(-y1 , deltah);
end

== matlab function Los_path_old/MATLAB Function1 ==
  data: CartPosError input; bodyPosError output; eta input
function bodyPosError = Rotation(CartPosError, eta)
    angle = eta(3);
    bodyPosError = zeros(4,1);
    rot = [cos(angle), -sin(angle)
            sin(angle), cos(angle)];

    bodyPosError(1:2) = rot' * CartPosError(1:2);
    bodyPosError(3:4) = CartPosError(3:4);
end

== matlab function Los_path_old/MATLAB Function9 ==
  data: p_pose_err input; depth_des input; err_pos output; psi_path input
function err_pos = psi_err(p_pose_err, depth_des, psi_path)
    err_pos = zeros(4,1);
    err_pos(3) = psi_path - p_pose_err(3);
    err_pos(4) = depth_des - p_pose_err(4);
end

== matlab function Los_path_old/PID Controller Circo/Depth PID/MATLAB Function1 ==
  data: u_cart input; bodyPosError output; eta input
function bodyPosError = Rotation(u_cart, eta)
    angle = eta(3);
    bodyPosError = zeros(4,1);
    rot = [cos(angle), -sin(angle)
            sin(angle), cos(angle)];

    bodyPosError(1:2) = rot' * u_cart(1:2);
    bodyPosError(3:4) = u_cart(3:4);
end

== matlab function Los_path_old/MATLAB Function5 ==
  data: x_dot input; tau input; tau0 input; x_dotdot output; speed0 input
function x_dotdot = vehicle_dynamics_matrix(x_dot, tau, tau0, speed0)
    % updated to medusa model
    m = 30;
    I = 4.14;

    % Added mass
    tau_a = [-25; -2.325; -8.690; -19.4311]; % kl_dot

    % Restoring forces
    tau_r = [-0.2; -55.117; -4.14; 33.6804]; % kl

    % Hydrodynamic forces
    tau_d = [-19.5; -147.9; -6.23; -89.4105]; % kl_modl

    % Virtual mass
    mv = [m; m; I; m] - tau_a;

    % Dissatipative forces
    dv = -tau_r - 2*tau_d .* abs(speed0);

    delta = x_dot - speed0;

    % Accelerations
    % 3 DOF MODEL Linearized
    x_dotdot = zeros(4,1);
    tau(2) = 0;
    x_dotdot(1) = (tau(1) - tau0(1) - dv(1)*delta(1) + mv(2)*speed0(2)*delta(3) + mv(2)*speed0(3)*delta(2)) / mv(1); 
    x_dotdot(2) = (tau(2) - tau0(2) - dv(2)*delta(2) - mv(1)*speed0(1)*delta(3) - mv(1)*speed0(3)*delta(1)) / mv(2);
    x_dotdot(3) = (tau(3) - tau0(3) - dv(3)*delta(3) + (mv(1) - mv(2))*speed0(1)*delta(2) + (mv(1) - mv(2))*speed0(2)*delta(1)) / mv(3);
    % Considering also depth (heavy)
    x_dotdot(4) = (tau(4) - tau0(4) + dv(4)*delta(4)) / mv(4);
end

== matlab function Los_path_old/MATLAB Function12 ==
  data: m input; psi_p output
function psi_p = trajectory_orientation(m)
    psi_p = atan(m); % already in radiants
end
